simulink model "ModelloParametroNoto"  (R2025b)
settings: Solver=ode45  StartTime=0.0  StopTime=10  MaxStep=1e-3  RelTol=1e-3
values from neighbouring files (symbols this model uses):
  a = 5    [main.m]
  K = 2    [main.m]
settings Model: Creator=Armando  LastModifiedBy=Armando

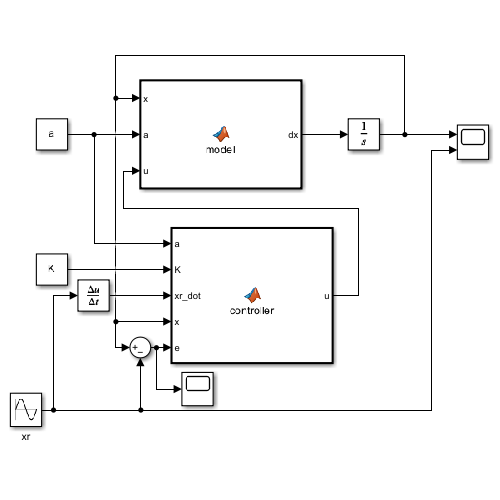
[thumbnail: Simulink's stored preview of the top-level diagram]
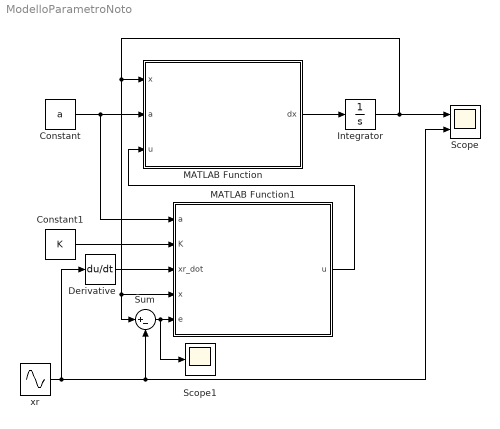
== system ModelloParametroNoto ==
  Constant : Constant  Value=a
  Constant1 : Constant  Value=K
  Derivative : Derivative
  Integrator : Integrator  InitialCondition=2
  MATLAB Function : MATLAB Function  TreatAsAtomicUnit=on
  MATLAB Function1 : MATLAB Function  TreatAsAtomicUnit=on
  Scope : Scope  NumInputPorts=2
      settings: ActiveDisplayYMinimum=-1.3749999148905223  ActiveDisplayYMaximum=2.3749999905433912
  Scope1 : Scope
      settings: ActiveDisplayYMinimum=-0.253261008364723  ActiveDisplayYMaximum=2.2503623342627468
  Sum : Sum  Inputs=|+-
  xr : Sin  SampleTime=0
  wires:
  MATLAB Function/1(dx) -> Integrator/1
  Integrator/1 -> Sum/1, MATLAB Function1/4(x), MATLAB Function/1(x), Scope/1
  Constant/1 -> MATLAB Function/2(a), MATLAB Function1/1(a)
  Constant1/1 -> MATLAB Function1/2(K)
  Sum/1 -> Scope1/1, MATLAB Function1/5(e)
  xr/1 -> Scope/2, Sum/2, Derivative/1
  MATLAB Function1/1(u) -> MATLAB Function/3(u)
  Derivative/1 -> MATLAB Function1/3(xr_dot)

== matlab function ModelloParametroNoto/MATLAB Function1 ==
  data: a input; u output; K input; xr_dot input; x input; e input
function u = controller(a,K,xr_dot,x,e)
u =  (- a*x) + xr_dot - (K * e);

== matlab function ModelloParametroNoto/MATLAB Function ==
  data: x input; a input; u input; dx output
function dx = model(x, a,u)
dx = a*x + u;
